simulink subsystem "bh_COMPONENT_wrap_angles"  (R2020a)
settings: Solver=VariableStepAuto  StartTime=0.0  StopTime=10.0  RelTol=1e-3
settings Model: Creator=bhorton  LastModifiedBy=bhorton

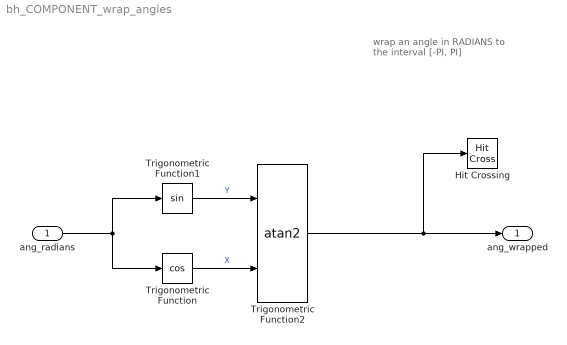
== system bh_COMPONENT_wrap_angles ==
  note: wrap an angle in RADIANS
      | to the interval [-PI, PI]
  ang_radians : Inport
  Hit Crossing : HitCross
  Trigonometric Function : Trigonometry  Operator=cos
  Trigonometric Function1 : Trigonometry
  Trigonometric Function2 : Trigonometry  Operator=atan2
  ang_wrapped : Outport
  wires:
  ang_radians/1 -> Trigonometric Function1/1, Trigonometric Function/1
  Trigonometric Function/1 -> Trigonometric Function2/2  "X"
  Trigonometric Function1/1 -> Trigonometric Function2/1  "Y"
  Trigonometric Function2/1 -> ang_wrapped/1, Hit Crossing/1
